simulink model "chema_tau"  (R2021b)
settings: Solver=VariableStepAuto  StartTime=0.0  StopTime=10.0  RelTol=1e-3
undefined symbols (not defined in the file): A, B, K
settings Model: Creator=osini  LastModifiedBy=osini

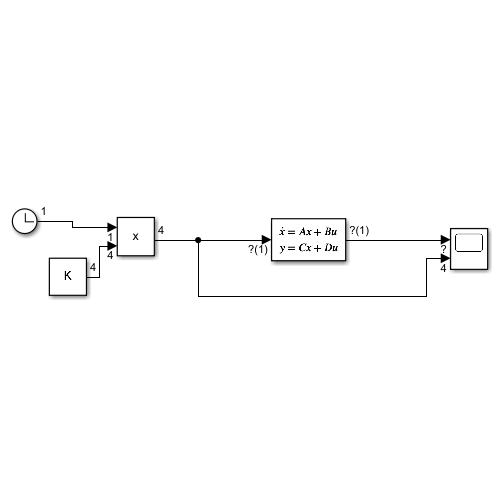
[thumbnail: Simulink's stored preview of the top-level diagram]
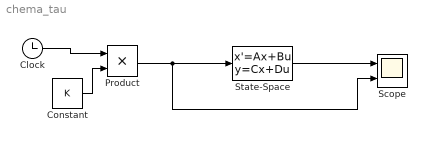
== system chema_tau ==
  Clock : Clock
  Constant : Constant  Value=K
  Product : Product
  Scope : Scope  NumInputPorts=2
  State-Space : StateSpace  A=A  B=B  C=[1 1 1 1]  D=0  InitialCondition=1
  wires:
  Product/1 -> State-Space/1, Scope/2
  Clock/1 -> Product/1
  Constant/1 -> Product/2
  State-Space/1 -> Scope/1
